simulink model "lqr_1dof_linear_force"  (R2017a)
settings: Solver=ode45  StartTime=0.0  StopTime=10  RelTol=1e-3
undefined symbols (not defined in the file): A, B, GoalPos, K, x0
settings Model: Creator=sansh  LastModifiedBy=Lucifer

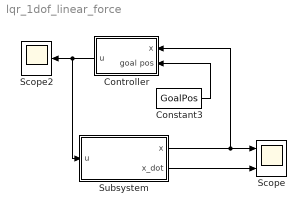
== system lqr_1dof_linear_force ==
  Constant3 : Constant  Value=GoalPos
  Controller : Subsystem
  Scope : Scope  NumInputPorts=2
  Scope2 : Scope
  Subsystem : Subsystem
  wires:
  Constant3/1 -> Controller/2(goal pos)
  Subsystem/2(x_dot) -> Scope/2
  Subsystem/1(x) -> Controller/1(x), Scope/1
  Controller/1(u) -> Subsystem/1(u), Scope2/1

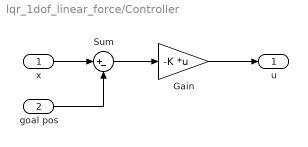
== system lqr_1dof_linear_force/Controller ==
  x : Inport
  goal pos : Inport  Port=2
  Gain : Gain  Gain=-K  Multiplication=Matrix(K*u)
  Sum : Sum  Inputs=|+-
  u : Outport
  wires:
  x/1 -> Sum/1
  Gain/1 -> u/1
  Sum/1 -> Gain/1
  goal pos/1 -> Sum/2

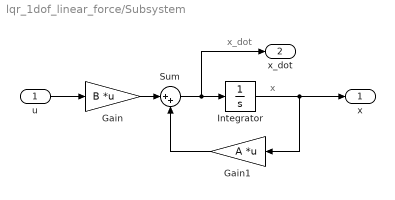
== system lqr_1dof_linear_force/Subsystem ==
  note: x_dot
  note: x
  u : Inport
  Gain : Gain  Gain=B  Multiplication=Matrix(K*u)
  Gain1 : Gain  Gain=A  Multiplication=Matrix(K*u)
  Integrator : Integrator  InitialCondition=x0
  Sum : Sum  Inputs=|++
  x : Outport
  x_dot : Outport  Port=2
  wires:
  Gain1/1 -> Sum/2
  Integrator/1 -> Gain1/1, x/1
  u/1 -> Gain/1
  Sum/1 -> x_dot/1, Integrator/1
  Gain/1 -> Sum/1
